simulink model "dc_motor"  (R2014a)
settings: Solver=ode45  StartTime=0.0  StopTime=5  RelTol=1e-3
settings Model: Creator=Divya M  LastModifiedBy=Divya M

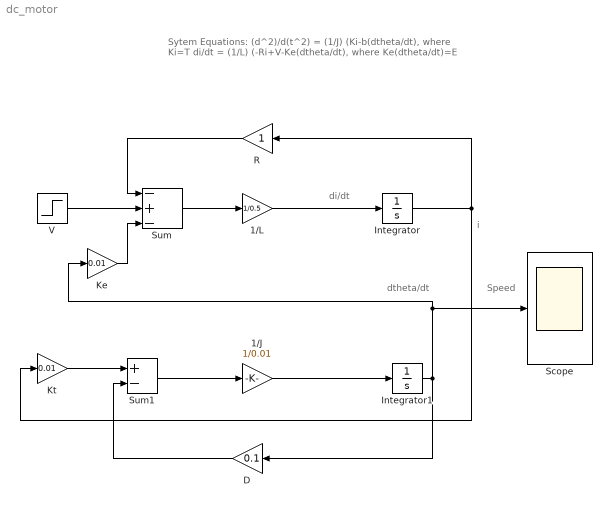
== system dc_motor ==
  note: Sytem Equations:
      |
      | (d^2)/d(t^2) = (1/J) (Ki-b(dtheta/dt), where Ki=T
      | di/dt = (1/L) (-Ri+V-Ke(dtheta/dt), where Ke(dtheta/dt)=E
  note: Speed
  note: dtheta/dt
  note: i
  note: di/dt
  1/J : Gain  Gain=1/0.01
  1/L : Gain  Gain=1/0.5
  D : Gain  Gain=0.1
  Integrator : Integrator
  Integrator1 : Integrator
  Ke : Gain  Gain=0.01
  Kt : Gain  Gain=0.01
  R : Gain
  Scope : Scope
      settings: YMin=-0.01  YMax=0.11
  Sum : Sum  Inputs=-+-
  Sum1 : Sum  Inputs=+-
  V : Step  SampleTime=0
  wires:
  V/1 -> Sum/2
  R/1 -> Sum/1
  Sum/1 -> 1/L/1
  1/L/1 -> Integrator/1
  Integrator/1 -> R/1, Kt/1
  Ke/1 -> Sum/3
  Kt/1 -> Sum1/1
  Sum1/1 -> 1/J/1
  1/J/1 -> Integrator1/1
  Integrator1/1 -> Ke/1, Scope/1, D/1
  D/1 -> Sum1/2
